simulink model "doc_audioscrambler"  (R2014a)
settings: Solver=FixedStepDiscrete  SolverMode=SingleTasking  StartTime=0.0  StopTime=inf  RelTol=1e-3
undefined symbols (not defined in the file or in its folder): commblksprivate, Info
libraries: commutil2 x4, commsequence2 x2, dspvision x1
settings Model: Creator=The MathWorks Inc.
settings SolverCC: InsertRTBMode=Auto
settings DataIOCC: SignalLoggingSaveFormat=ModelDataLogs
settings OptimizationCC: ExpressionDepthLimit=2147483647  InitFltsAndDblsToZero=on  EfficientMapNaN2IntZero=off
settings DebuggingCC: UnderspecifiedInitializationDetection=Classic  FcnCallInpInsideContextMsg=UseLocalSettings  StateNameClashWarn=warning  StrictBusMsg=Warning
settings HardwareCC: ProdHWDeviceType=ASIC/FPGA->ASIC/FPGA  TargetBitPerLong=64  TargetBitPerPointer=64  TargetLongLongMode=on  TargetEndianess=LittleEndian  TargetWordSize=64  TargetHWDeviceType=MATLAB Host  ProdEqTarget=off
settings GRTTargetCC: CombineOutputUpdateFcns=off  GRTInterface=on

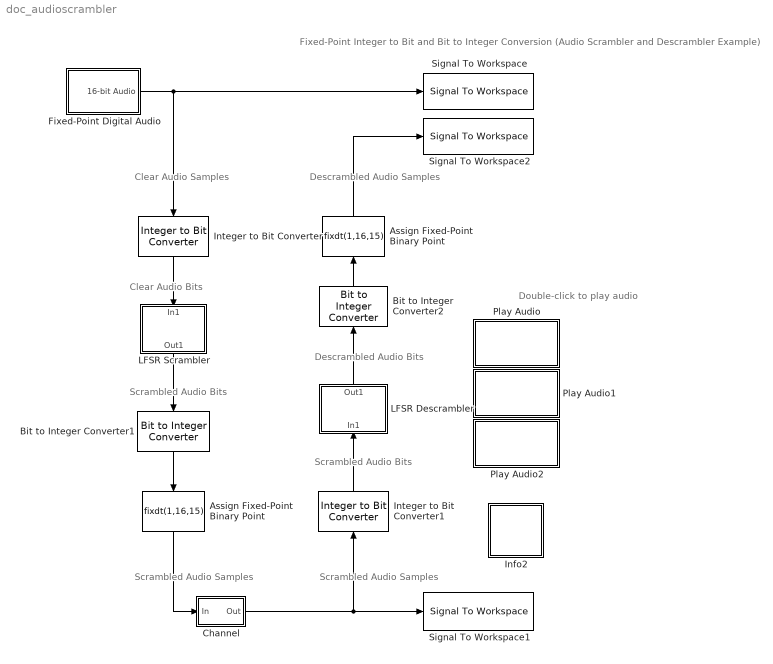
== system doc_audioscrambler ==
  note: Fixed-Point Integer to Bit and Bit to Integer Conversion
      | (Audio Scrambler and Descrambler Example)
  note: Scrambled
      | Audio
      | Samples
  note: Descrambled
      | Audio Samples
  note: Clear Audio
      | Samples
  note: Scrambled
      | Audio Bits
  note: Clear Audio
      | Bits
  note: Descrambled
      | Audio Bits
  note: Scrambled
      | Audio Bits
  note: Scrambled
      | Audio
      | Samples
  note: Double-click to
      | play audio
  Assign Fixed-Point Binary Point : DataTypeConversion  OutMin=-1  OutMax=(32767/32768)  OutDataTypeStr=fixdt(1,16,15)  ConvertRealWorld=Stored Integer (SI)
  Assign Fixed-Point Binary Point : DataTypeConversion  OutMin=-1  OutMax=(32767/32768)  OutDataTypeStr=fixdt(1,16,15)  ConvertRealWorld=Stored Integer (SI)
  Bit to Integer Converter1 : commutil2/Bit to Integer Converter  nbits=16  bitOrder=MSB first  signedOutputValues=Signed  outDtype=Inherit via internal rule  outDtypeSigned=Inherit via internal rule
  Bit to Integer Converter2 : commutil2/Bit to Integer Converter  nbits=16  bitOrder=MSB first  signedOutputValues=Signed  outDtype=Inherit via internal rule  outDtypeSigned=Inherit via internal rule
  Channel : Subsystem
  Fixed-Point Digital Audio : Subsystem
  Info2 : Subsystem  AncestorBlock=commblksprivate/Info  mask(Info){}
      settings: OpenFcn=helpview([docroot '/toolbox/comm/comm.map'], 'doc_audioscrambler')
      mask Display: disp('Info')
  Integer to Bit Converter : commutil2/Integer to Bit Converter  nbits=16  signedInputValues=Signed  bitOrder=MSB first  outDtype=Inherit via internal rule
  Integer to Bit Converter1 : commutil2/Integer to Bit Converter  nbits=16  signedInputValues=Signed  bitOrder=MSB first  outDtype=Inherit via internal rule
  LFSR Descrambler : Subsystem
      mask Display: disp('LFSR\nDescrambler');
  LFSR Scrambler : Subsystem
      mask Display: disp('LFSR\nScrambler');
  Play Audio : Subsystem
      settings: OpenFcn=|
      | if exist('clearAudio','var')
      |    sound(clearAudio, 22050);
      | end
      mask Display: disp('Play Audio:\nClear');
  Play Audio1 : Subsystem
      settings: OpenFcn=|
      | if exist('scrambledAudio','var')
      |    sound(scrambledAudio, 22050);
      | end
      mask Display: disp('Play Audio:\nScrambled');
  Play Audio2 : Subsystem
      settings: OpenFcn=|
      | if exist('descrambledAudio','var')
      |    sound(descrambledAudio, 22050);
      | end
      mask Display: disp('Play Audio:\nDescrambled');
  Signal To Workspace : SignalToWorkspace  VariableName=clearAudio
      settings: CopyFcn=dspblkcopystw(gcbh);  Save2DSignal=Inherit from input (this choice will be removed - see release notes)
  Signal To Workspace1 : SignalToWorkspace  VariableName=scrambledAudio
      settings: CopyFcn=dspblkcopystw(gcbh);  Save2DSignal=Inherit from input (this choice will be removed - see release notes)
  Signal To Workspace2 : SignalToWorkspace  VariableName=descrambledAudio
      settings: CopyFcn=dspblkcopystw(gcbh);  Save2DSignal=Inherit from input (this choice will be removed - see release notes)
  wires:
  Fixed-Point Digital Audio/1(16-bit Audio) -> Integer to Bit Converter/1, Signal To Workspace/1
  Integer to Bit Converter/1 -> LFSR Scrambler/1(In1)
  Bit to Integer Converter1/1 -> Assign Fixed-Point Binary Point/1
  Assign Fixed-Point Binary Point/1 -> Channel/1(In)
  Integer to Bit Converter1/1 -> LFSR Descrambler/1(In1)
  LFSR Scrambler/1(Out1) -> Bit to Integer Converter1/1
  LFSR Descrambler/1(Out1) -> Bit to Integer Converter2/1
  Bit to Integer Converter2/1 -> Assign Fixed-Point Binary Point/1
  Assign Fixed-Point Binary Point/1 -> Signal To Workspace2/1
  Channel/1(Out) -> Signal To Workspace1/1, Integer to Bit Converter1/1

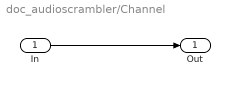
== system doc_audioscrambler/Channel ==
  In : Inport
  Out : Outport
  wires:
  In/1 -> Out/1

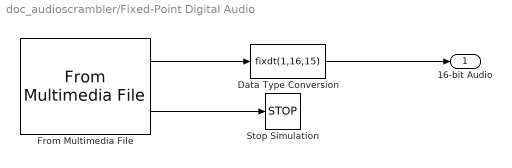
== system doc_audioscrambler/Fixed-Point Digital Audio ==
  Data Type Conversion : DataTypeConversion  OutMin=-1  OutMax=(32767/32768)  OutDataTypeStr=fixdt(1,16,15)  ConvertRealWorld=Stored Integer (SI)
  From Multimedia File : dspvision/From Multimedia File  inputFilename=speech_dft.avi  loop=on  numPlays=1  outputStreams=Audio only  videoDataType=single  audioDataType=int16  inheritSampleTime=on  userDefinedSampleTime=1/30  noAudioOutput=off  isIntensityVideo=off  fourcc=RGB  colorVideoFormat=Separate color signals  outputEOF=on  dataOrg=Column-major  audioFrameSize=1024  computeAudioFrameSize=off  outSamplingMode=Frame based
  Stop Simulation : Stop
  16-bit Audio : Outport
  wires:
  From Multimedia File/1 -> Data Type Conversion/1
  From Multimedia File/2 -> Stop Simulation/1
  Data Type Conversion/1 -> 16-bit Audio/1

== system doc_audioscrambler/Info2 ==

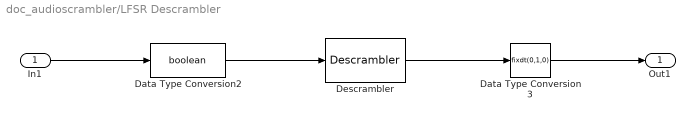
== system doc_audioscrambler/LFSR Descrambler ==
  In1 : Inport
  Data Type Conversion2 : DataTypeConversion  OutMin=0  OutMax=1  OutDataTypeStr=boolean
  Data Type Conversion3 : DataTypeConversion  OutMin=0  OutMax=1  OutDataTypeStr=fixdt(0,1,0)
  Descrambler : commsequence2/Descrambler  M=2  poly=[1 1 1 0 1]  ini_sta=[0 1 1 0]
  Out1 : Outport
  wires:
  Descrambler/1 -> Data Type Conversion3/1
  Data Type Conversion2/1 -> Descrambler/1
  In1/1 -> Data Type Conversion2/1
  Data Type Conversion3/1 -> Out1/1

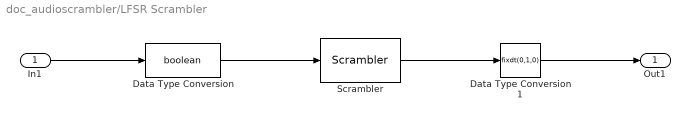
== system doc_audioscrambler/LFSR Scrambler ==
  In1 : Inport
  Data Type Conversion : DataTypeConversion  OutMin=0  OutMax=1  OutDataTypeStr=boolean
  Data Type Conversion1 : DataTypeConversion  OutMin=0  OutMax=1  OutDataTypeStr=fixdt(0,1,0)
  Scrambler : commsequence2/Scrambler  M=2  poly=[1 1 1 0 1]  ini_sta=[0 1 1 0]
  Out1 : Outport
  wires:
  Scrambler/1 -> Data Type Conversion1/1
  Data Type Conversion/1 -> Scrambler/1
  In1/1 -> Data Type Conversion/1
  Data Type Conversion1/1 -> Out1/1

== system doc_audioscrambler/Play Audio ==
  note: This is an empty subsystem.

== system doc_audioscrambler/Play Audio1 ==
  note: This is an empty subsystem.

== system doc_audioscrambler/Play Audio2 ==
  note: This is an empty subsystem.
